simulink model "sampleModel74"  (R2021b)
settings: Solver=VariableStepAuto  StartTime=0.0  StopTime=10.0  RelTol=1e-3
undefined symbols (not defined in the file or in its folder): magnitude, Newton, Raphson
libraries: simulink x10, slpidlib x2
settings Model: Creator=user  LastModifiedBy=user

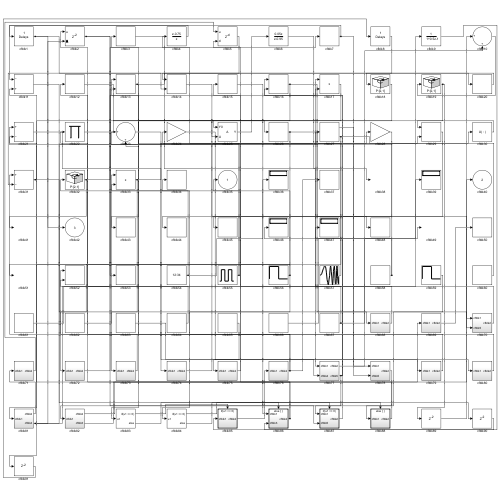
[thumbnail: Simulink's stored preview of the top-level diagram]
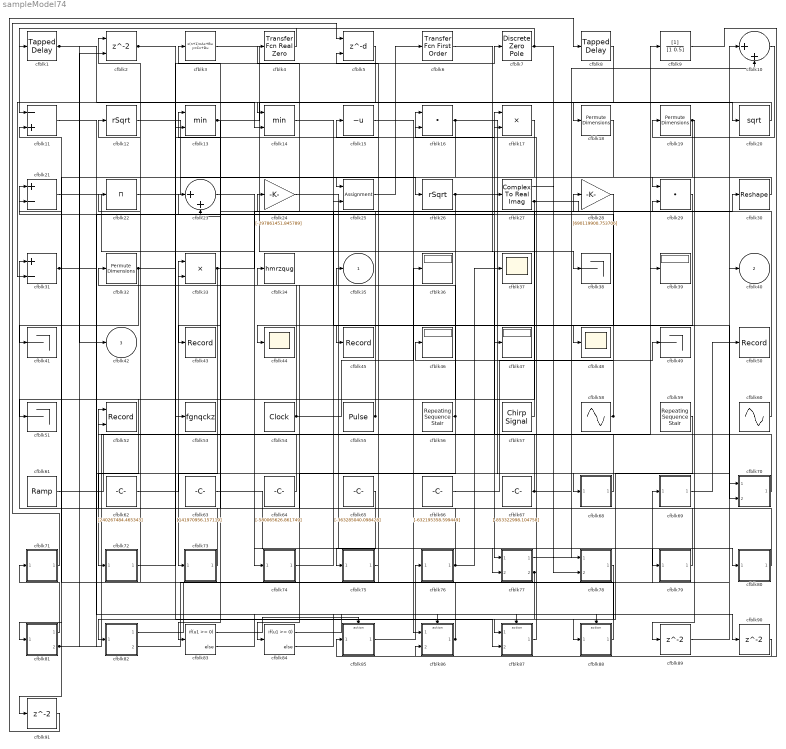
== system sampleModel74 ==
  cfblk1 : simulink/Discrete/Tapped Delay  vinit=0.0  samptime=-1  NumDelays=1  DelayOrder=Oldest  includeCurrent=off
  cfblk10 : Sum  Inputs=|++
  cfblk11 : Sum  Inputs=-+
  cfblk12 : Sqrt  Operator=rSqrt  AlgorithmType=Newton-Raphson  SaturateOnIntegerOverflow=on
  cfblk13 : MinMax  Inputs=2
  cfblk14 : MinMax  Inputs=2
  cfblk15 : UnaryMinus
  cfblk16 : DotProduct  InputSameDT=on  OutDataTypeStr=Inherit: Inherit via internal rule
  cfblk17 : Product
  cfblk18 : PermuteDimensions
  cfblk19 : PermuteDimensions
  cfblk2 : Delay  ShowEnablePort=on  SampleTime=1
      settings: InputPortMap=u0,e6
  cfblk20 : Sqrt  SaturateOnIntegerOverflow=on
  cfblk21 : Sum  Inputs=+-
  cfblk22 : Product  Inputs=*
  cfblk23 : Sum  Inputs=|++
  cfblk24 : Gain  Gain=[-297861451.845789]
  cfblk25 : Assignment  DiagnosticForDimensions=Warning  IndexOptions=Index vector (dialog)  Indices=1  OutputSizes=1
  cfblk26 : Sqrt  Operator=rSqrt  AlgorithmType=Newton-Raphson  SaturateOnIntegerOverflow=on
  cfblk27 : ComplexToRealImag
  cfblk28 : Gain  Gain=[690119900.753706]
  cfblk29 : DotProduct  InputSameDT=on  OutDataTypeStr=Inherit: Inherit via internal rule
  cfblk3 : DiscreteStateSpace
  cfblk30 : Reshape
  cfblk31 : Sum  Inputs=+-
  cfblk32 : PermuteDimensions
  cfblk33 : Product  Inputs=**
  cfblk34 : ToWorkspace  VariableName=hmrzqug  SaveFormat=Timeseries  SampleTime=-1
  cfblk{36,39,46..47} (4 alike) : Display
  cfblk37 : Scope
  cfblk{38,41,49,51} (4 alike) : Terminator
  cfblk4 : simulink/Discrete/Transfer Fcn Real Zero  ZeroZ=0.75  ICPrevInput=0.0  DoSatur=off
      settings: SourceProductBaseCode=SL
  cfblk43 : Record  FileSettingsInternal="{\"entries\":[{\"content\":{\"excelSettings\":{\"content\":{},\"type\":\"Streamout.ExcelSettings\"}},\"type\":\"Streamout.FileSettingStorage\",\"uuid\":\"48ba1b95-7696-4fb7-898a-d0dd139d0650\"}],\"packageUris\":[\"http://schema.mathworks.com/mf0/streamout_blocks/R2020a\"],\"version\":\"1.0\"}"  SignalsInternal="{\"entries\":[{\"content\":{\"signals\":[{\"content\":{\"blockPath\":[\"sampleModel74/cfblk43\"],\"channel\":[],\"dimensions\":[1,1],\"domain\":\"sampleModel74/cfblk43\",\"lineColor\":\"#edb120\",\"plots\":[1],\"port\":1,\"sid\":[\"\"],\"signalID\":2737,\"signalName\":\"cfblk17\"},\"type\":\"RecordBlkView.Signal\",\"uuid\":\"e86d3584-fb59-4afd-a1db-0bd2ffc62248\"}]},\"type\":\"RecordBlkView.InputSignals\",\"uuid\":\"38ef3183-be6e-4a9e-be3e-a4fb90b5b1f9\"}],\"packageUris\":[\"http://schema.mathworks.com/mf0/streamout_blocks/R2020a\"],\"version\":\"1.0\"}"  VisualizationBindings="{\"sparklinesplugin\":{\"info\":[{\"bindingParametersList\":[],\"subplotID\":1}]}}"
  cfblk44 : Scope
  cfblk45 : Record  FileSettingsInternal="{\"entries\":[{\"content\":{\"excelSettings\":{\"content\":{},\"type\":\"Streamout.ExcelSettings\"}},\"type\":\"Streamout.FileSettingStorage\",\"uuid\":\"c0c04c6a-9287-4ca5-a954-90f3d465e295\"}],\"packageUris\":[\"http://schema.mathworks.com/mf0/streamout_blocks/R2020a\"],\"version\":\"1.0\"}"  SignalsInternal="{\"entries\":[{\"content\":{\"signals\":[{\"content\":{\"blockPath\":[\"sampleModel74/cfblk45\"],\"channel\":[],\"dimensions\":[1],\"domain\":\"sampleModel74/cfblk45\",\"lineColor\":\"#7e2f8e\",\"plots\":[1],\"port\":1,\"sid\":[\"\"],\"signalID\":2741,\"signalName\":\"cfblk28\"},\"type\":\"RecordBlkView.Signal\",\"uuid\":\"fff33049-bbd2-4e7c-9b44-5c2925b8b3c0\"}]},\"type\":\"RecordBlkView.InputSignals\",\"uuid\":\"e4e584d3-6e89-4657-a415-00abe31742ed\"}],\"packageUris\":[\"http://schema.mathworks.com/mf0/streamout_blocks/R2020a\"],\"version\":\"1.0\"}"  VisualizationBindings="{\"sparklinesplugin\":{\"info\":[{\"bindingParametersList\":[],\"subplotID\":1}]}}"
  cfblk48 : Scope
  cfblk5 : Delay  DelayLengthSource=Input port  SampleTime=1
      settings: InputPortMap=u0,p1
  cfblk50 : Record  FileSettingsInternal="{\"entries\":[{\"content\":{\"excelSettings\":{\"content\":{},\"type\":\"Streamout.ExcelSettings\"}},\"type\":\"Streamout.FileSettingStorage\",\"uuid\":\"2063bf91-ee10-44c6-85e7-3db64ce144e7\"}],\"packageUris\":[\"http://schema.mathworks.com/mf0/streamout_blocks/R2020a\"],\"version\":\"1.0\"}"  SignalsInternal="{\"entries\":[{\"content\":{\"signals\":[{\"content\":{\"blockPath\":[\"sampleModel74/cfblk50\"],\"channel\":[],\"dimensions\":[1],\"domain\":\"sampleModel74/cfblk50\",\"lineColor\":\"#77ac30\",\"plots\":[1],\"port\":1,\"sid\":[\"\"],\"signalID\":2745,\"signalName\":\"cfblk69\"},\"type\":\"RecordBlkView.Signal\",\"uuid\":\"c73e1d6d-ec7e-4053-a185-d07a06e2b1ae\"}]},\"type\":\"RecordBlkView.InputSignals\",\"uuid\":\"2d8ce3cf-72b1-4d47-bc01-c7806f849a67\"}],\"packageUris\":[\"http://schema.mathworks.com/mf0/streamout_blocks/R2020a\"],\"version\":\"1.0\"}"  VisualizationBindings="{\"sparklinesplugin\":{\"info\":[{\"bindingParametersList\":[],\"subplotID\":1}]}}"
  cfblk52 : Record  FileSettingsInternal="{\"entries\":[{\"content\":{\"excelSettings\":{\"content\":{},\"type\":\"Streamout.ExcelSettings\"}},\"type\":\"Streamout.FileSettingStorage\",\"uuid\":\"a33d63da-2fbc-4813-9a5f-8919b3ff38c5\"}],\"packageUris\":[\"http://schema.mathworks.com/mf0/streamout_blocks/R2020a\"],\"version\":\"1.0\"}"  Layout=[1 1]  SignalsInternal="{\"entries\":[{\"content\":{\"signals\":[{\"content\":{\"blockPath\":[\"sampleModel74/cfblk52\"],\"channel\":[],\"dimensions\":[1],\"domain\":\"sampleModel74/cfblk52\",\"lineColor\":\"#a2142f\",\"plots\":[1],\"port\":1,\"sid\":[\"\"],\"signalID\":2749,\"signalName\":\"cfblk73\"},\"type\":\"RecordBlkView.Signal\",\"uuid\":\"3106f9a6-1d98-4c48-b4a9-0628818cd6a2\"},{\"content\":{\"blockPath\":[\"sampleModel74/cfblk52\"],\"channel\":[],\"dimensions\":[1],\"domain\":\"sampleModel74/cfblk52\",\"lineColor\":\"#139fff\",\"plots\":[1],\"port\":2,\"sid\":[\"\"],\"signalID\":2753,\"signalName\":\"cfblk64\"},\"type\":\"RecordBlkView.Signal\",\"uuid\":\"3007701b-6436-4cea-b82a-5ba8fd36c4e2\"}]},\"type\":\"RecordBlkView.InputSignals\",\"uuid\":\"9f57cf0e-22d1-4040-b944-b37ea4da367a\"}],\"packageUris\":[\"http://schema.mathworks.com/mf0/streamout_blocks/R2020a\"],\"version\":\"1.0\"}"  VisualizationBindings="{\"xyplotplugin\":{\"info\":[{\"series\":[{\"bindingParametersList\":[{\"parameter\":\"X-Axis\",\"signalID\":2749,\"signalName\":\"cfblk73\"},{\"parameter\":\"Y-Axis\",\"signalID\":2753,\"signalName\":\"cfblk64\"}],\"seriesID\":56445}],\"subplotID\":1}]}}"  CompatibilityTag=XY
  cfblk53 : ToWorkspace  VariableName=fgnqckz  SaveFormat=Timeseries  SampleTime=-1
  cfblk54 : DigitalClock
  cfblk55 : DiscretePulseGenerator  PulseType=Time based  Amplitude=[301093662.355844]  Period=[78291214.877593]  PulseWidth=5  PhaseDelay=[1.000000]
  cfblk56 : simulink/Sources/Repeating Sequence Stair  OutValues=[-38877685.461158, -866960158.323522]  tsamp=-1  OutMin=[]  OutMax=[]  OutDataTypeStr=double  OutputDataTypeScalingMode=double  OutDataType=fixdt(0,8)  ConRadixGroup=Best Precision: Vector-wise  OutScaling=2^-12
  cfblk57 : simulink/Sources/Chirp Signal  f1=[-130713625.876900]  T=[92266406.941991]  f2=[714551221.409625]
  cfblk58 : Sin  Amplitude=[-215573379.116947]  Bias=[658746098.891417]  SampleTime=0
  cfblk59 : simulink/Sources/Repeating Sequence Stair  OutValues=[-482847382.722123, -898676029.322696]  tsamp=-1  OutMin=[]  OutMax=[]  OutDataTypeStr=double  OutputDataTypeScalingMode=double  OutDataType=fixdt(0,8)  ConRadixGroup=Best Precision: Vector-wise  OutScaling=2^-12
  cfblk6 : simulink/Discrete/Transfer Fcn First Order  PoleZ=0.95  ICPrevOutput=0.0  DoSatur=off
  cfblk60 : Sin  Amplitude=[827954509.071652]  Bias=[417393928.339158]  SampleTime=0
  cfblk61 : simulink/Sources/Ramp  slope=[3672.630180]  start=[38.252533]  InitialOutput=[-938336.900996]
  cfblk62 : Constant  Value=[240267484.465343]  SampleTime=1
  cfblk63 : Constant  Value=[141970956.157119]  SampleTime=1
  cfblk64 : Constant  Value=[-580065626.861749]  SampleTime=1
  cfblk65 : Constant  Value=[-363285040.098428]  SampleTime=1
  cfblk66 : Constant  Value=[-632195358.599449]  SampleTime=1
  cfblk67 : Constant  Value=[-853322998.104758]  SampleTime=1
  cfblk68 : Subsystem
  cfblk69 : Subsystem
  cfblk7 : DiscreteZeroPole  Poles=[0 0.5]  Gain=1
  cfblk70 : Subsystem
  cfblk71 : Subsystem
  cfblk72 : Subsystem
  cfblk73 : Subsystem
  cfblk74 : Subsystem
  cfblk75 : Subsystem
  cfblk76 : Subsystem
  cfblk77 : Subsystem
  cfblk78 : Subsystem
  cfblk79 : Subsystem
  cfblk8 : simulink/Discrete/Tapped Delay  vinit=0.0  samptime=-1  NumDelays=1  DelayOrder=Oldest  includeCurrent=off
  cfblk80 : Subsystem
  cfblk81 : Subsystem
  cfblk82 : Subsystem
  cfblk83 : If  IfExpression=u1 >= 0  SampleTime=1
  cfblk84 : If  IfExpression=u1 >= 0  SampleTime=1
  cfblk85 : Subsystem  TreatAsAtomicUnit=on
  cfblk86 : Subsystem  TreatAsAtomicUnit=on
  cfblk87 : Subsystem  TreatAsAtomicUnit=on
  cfblk88 : Subsystem  TreatAsAtomicUnit=on
  cfblk89 : Delay  SampleTime=1
  cfblk9 : DiscreteFilter  SampleTime=1
  cfblk90 : Delay  SampleTime=1
  cfblk91 : Delay  SampleTime=1
  cfblk35 : Outport
  cfblk40 : Outport  Port=2
  cfblk42 : Outport  Port=3
  wires:
  cfblk25/1 -> cfblk6/1
  cfblk54/1 -> cfblk32/1, cfblk36/1
  cfblk82/1(cfblk2) -> cfblk69/1(cfblk1)
  cfblk73/1(cfblk2) -> cfblk52/1
  cfblk3/1 -> cfblk77/1(cfblk1)
  cfblk27/1 -> cfblk78/1(cfblk1)
  cfblk1/1 -> cfblk42/1, cfblk14/2
  cfblk33/1 -> cfblk73/1(cfblk1), cfblk29/2
  cfblk57/1 -> cfblk24/1
  cfblk65/1 -> cfblk75/1(cfblk1)
  cfblk85/1(cfblk2) -> cfblk76/1(cfblk1)
  cfblk29/1 -> cfblk44/1
  cfblk16/1 -> cfblk68/1(cfblk1), cfblk83/1
  cfblk74/1(cfblk2) -> cfblk28/1
  cfblk64/1 -> cfblk52/2
  cfblk12/1 -> cfblk25/1
  cfblk76/1(cfblk2) -> cfblk31/1, cfblk34/1, cfblk37/1
  cfblk4/1 -> cfblk11/1
  cfblk23/1 -> cfblk77/2(cfblk4)
  cfblk75/1(cfblk2) -> cfblk15/1
  cfblk21/1 -> cfblk74/1(cfblk1)
  cfblk67/1 -> cfblk49/1, cfblk5/2
  cfblk13/1 -> cfblk20/1, cfblk23/2
  cfblk10/1 -> cfblk19/1
  cfblk8/1 -> cfblk18/1
  cfblk66/1 -> cfblk39/1
  cfblk56/1 -> cfblk33/1, cfblk84/1, cfblk51/1
  cfblk15/1 -> cfblk86/1(cfblk1)
  cfblk24/1 -> cfblk80/1(cfblk1)
  cfblk58/1 -> cfblk46/1, cfblk23/1
  cfblk55/1 -> cfblk4/1, cfblk21/2
  cfblk28/1 -> cfblk45/1
  cfblk68/1(cfblk2) -> cfblk17/1
  cfblk27/2 -> cfblk30/1, cfblk72/1(cfblk1)
  cfblk60/1 -> cfblk3/1
  cfblk87/1(cfblk2) -> cfblk47/1
  cfblk81/1(cfblk2) -> cfblk71/1(cfblk1)
  cfblk62/1 -> cfblk33/2
  cfblk17/1 -> cfblk43/1
  cfblk19/1 -> cfblk25/2, cfblk89/1
  cfblk20/1 -> cfblk14/1
  cfblk79/1(cfblk2) -> cfblk13/1
  cfblk5/1 -> cfblk31/2
  cfblk71/1(cfblk2) -> cfblk5/1
  cfblk61/1 -> cfblk9/1
  cfblk14/1 -> cfblk48/1
  cfblk78/1(cfblk2) -> cfblk87/1(cfblk1)
  cfblk22/1 -> cfblk26/1
  cfblk31/1 -> cfblk11/2, cfblk90/1
  cfblk7/1 -> cfblk1/1, cfblk78/2(cfblk5)
  cfblk69/1(cfblk2) -> cfblk50/1
  cfblk32/1 -> cfblk17/2, cfblk41/1
  cfblk81/2(cfblk4) -> cfblk13/2, cfblk27/1, cfblk2/2
  cfblk63/1 -> cfblk79/1(cfblk1)
  cfblk72/1(cfblk2) -> cfblk7/1
  cfblk59/1 -> cfblk88/1(cfblk1)
  cfblk88/1(cfblk2) -> cfblk35/1
  cfblk26/1 -> cfblk70/1(cfblk1), cfblk81/1(cfblk1)
  cfblk70/1(cfblk2) -> cfblk2/1
  cfblk2/1 -> cfblk53/1, cfblk87/2(cfblk5)
  cfblk77/1(cfblk2) -> cfblk10/2
  cfblk30/1 -> cfblk29/1
  cfblk6/1 -> cfblk38/1
  cfblk82/2(cfblk3) -> cfblk40/1
  cfblk80/1(cfblk2) -> cfblk22/1
  cfblk86/1(cfblk2) -> cfblk12/1, cfblk21/1
  cfblk77/2(cfblk5) -> cfblk82/1(cfblk1), cfblk16/1, cfblk16/2
  cfblk9/1 -> cfblk86/2(cfblk3)
  cfblk11/1 -> cfblk70/2(cfblk5)
  cfblk83/1 -> cfblk85/Action
  cfblk83/2 -> cfblk86/Action
  cfblk84/1 -> cfblk87/Action
  cfblk84/2 -> cfblk88/Action
  cfblk89/1 -> cfblk10/1
  cfblk90/1 -> cfblk85/1(cfblk1)
  cfblk18/1 -> cfblk91/1
  cfblk91/1 -> cfblk8/1

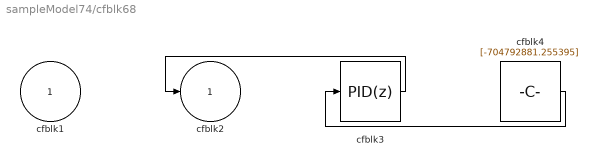
== system sampleModel74/cfblk68 ==
  cfblk1 : Inport
  cfblk3 : slpidlib/PID Controller  Controller=PID  Form=Parallel  TimeDomain=Discrete-time  UseExternalTs=off  SampleTime=1  IntegratorMethod=Forward Euler  FilterMethod=Forward Euler  ControllerParametersSource=internal  P=1  I=1  D=0  UseFilter=on  N=100  TunerSelectOption=Transfer Function Based (PID Tuner App)  InitialConditionSource=internal  InitialConditionForIntegrator=0  InitialConditionForFilter=0  DifferentiatorICPrevScaledInput=0  ExternalReset=none  TrackingMode=off  Kt=1  LimitOutput=off  SatLimitsSource=internal  UpperSaturationLimit=inf  LowerSaturationLimit=-inf  LinearizeAsGain=off  AntiWindupMode=none  Kb=1  POutMin=[]  POutMax=[]  IOutMin=[]  IOutMax=[]  DOutMin=[]  DOutMax=[]  NOutMin=[]  NOutMax=[]  SumOutMin=[]  SumOutMax=[]  SaturationOutMin=[]  SaturationOutMax=[]  PParamMin=[]  PParamMax=[]  IParamMin=[]  IParamMax=[]  DParamMin=[]  DParamMax=[]  NParamMin=[]  NParamMax=[]  KbParamMin=[]  KbParamMax=[]  KtParamMin=[]  KtParamMax=[]  KbOutMin=[]  KbOutMax=[]  KtOutMin=[]  KtOutMax=[]  IntegratorOutMin=[]  IntegratorOutMax=[]  FilterOutMin=[]  FilterOutMax=[]  SumI1OutMin=[]  SumI1OutMax=[]  SumI2OutMin=[]  SumI2OutMax=[]  SumI3OutMin=[]  SumI3OutMax=[]  SumI4OutMin=[]  SumI4OutMax=[]  SumDOutMin=[]  SumDOutMax=[]  DifferentiatorOutMin=[]  DifferentiatorOutMax=[]  FilterDiffOutCoefMin=[]  FilterDiffOutCoefMax=[]  ReciprocalOutMin=[]  ReciprocalOutMax=[]  SumDenOutMin=[]  SumDenOutMax=[]  SumNumOutMin=[]  SumNumOutMax=[]  DivideOutMin=[]  DivideOutMax=[]  UdiffTsProdOutMin=[]  UdiffTsProdOutMax=[]  NTsProdOutMin=[]  NTsProdOutMax=[]  UintegralTsProdOutMin=[]  UintegralTsProdOutMax=[]  UngainTsProdOutMin=[]  UngainTsProdOutMax=[]  IntegratorContinuousStateAttributes=''  IntegratorStateMustResolveToSignalObject=off  IntegratorRTWStateStorageClass=Auto  FilterContinuousStateAttributes=''  FilterStateMustResolveToSignalObject=off  FilterRTWStateStorageClass=Auto  ParallelPVariant=InternalParameters  IdealPVariant=Disabled  IVariant=InternalParameters  DVariant=InternalParameters  IntegratorVariant=Discrete  SatVariant=Disabled  AWVariant=Passthrough  PCopyVariant=Disabled  TRVariant=Disabled  FdbkBlocksVariant=Forward  IdealPFdbkVariant=Disabled  SatFdbkVariant=Disabled  DerivativeFilterVariant=ForwardEulerFilter  NVariant=InternalParameters  NCopyVariant=Disabled  FilterICVariant=InternalICsFilter  IntegratorICVariant=InternalICs  ExternalResetVariant=Disabled  TRSumVariant=Passthrough  SumFdbkVariant=Disabled  SumVariant=Sum_PID  TsampFilterVariant=InternalTs  TsampNgainVariant=Passthrough  TsampIntegralVariant=Passthrough  ExternalSaturationOutDataTypeStr=Inherit: Same as second input
  cfblk4 : Constant  Value=[-704792881.255395]  SampleTime=1
  cfblk2 : Outport
  wires:
  cfblk3/1 -> cfblk2/1
  cfblk4/1 -> cfblk3/1

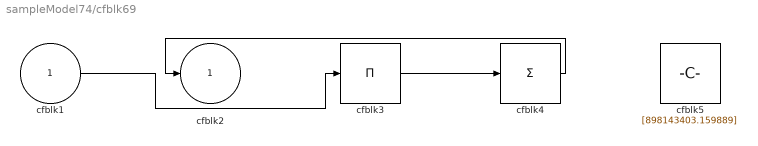
== system sampleModel74/cfblk69 ==
  cfblk1 : Inport
  cfblk3 : Product  Inputs=*
  cfblk4 : Sum  Inputs=+
  cfblk5 : Constant  Value=[898143403.159889]  SampleTime=1
  cfblk2 : Outport
  wires:
  cfblk3/1 -> cfblk4/1
  cfblk4/1 -> cfblk2/1
  cfblk1/1 -> cfblk3/1

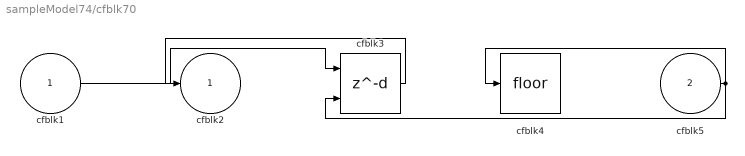
== system sampleModel74/cfblk70 ==
  cfblk1 : Inport
  cfblk5 : Inport  Port=2
  cfblk3 : Delay  DelayLengthSource=Input port  SampleTime=1
      settings: InputPortMap=u0,p1
  cfblk4 : Rounding
  cfblk2 : Outport
  wires:
  cfblk1/1 -> cfblk3/1
  cfblk5/1 -> cfblk3/2, cfblk4/1
  cfblk3/1 -> cfblk2/1

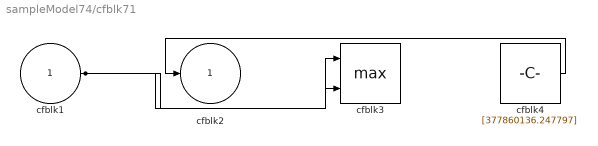
== system sampleModel74/cfblk71 ==
  cfblk1 : Inport
  cfblk3 : MinMax  Function=max  Inputs=2
  cfblk4 : Constant  Value=[377860136.247797]  SampleTime=1
  cfblk2 : Outport
  wires:
  cfblk4/1 -> cfblk2/1
  cfblk1/1 -> cfblk3/1, cfblk3/2

== system sampleModel74/cfblk72 ==
  cfblk1 : Inport
  cfblk3 : Constant  Value=[711047565.909843]  SampleTime=1
  cfblk2 : Outport
  wires:
  cfblk1/1 -> cfblk2/1

== system sampleModel74/cfblk73 ==
  cfblk1 : Inport
  cfblk3 : Constant  Value=[885206688.060875]  SampleTime=1
  cfblk2 : Outport
  wires:
  cfblk1/1 -> cfblk2/1

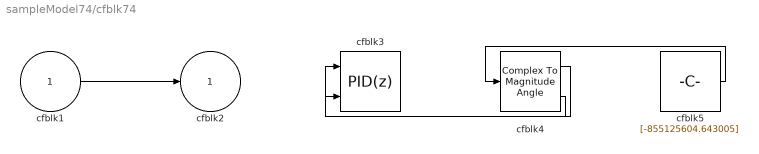
== system sampleModel74/cfblk74 ==
  cfblk1 : Inport
  cfblk3 : slpidlib/PID Controller (2DOF)  Controller=PID  Form=Parallel  TimeDomain=Discrete-time  UseExternalTs=off  SampleTime=1  IntegratorMethod=Forward Euler  FilterMethod=Forward Euler  ControllerParametersSource=internal  P=1  I=1  D=0  UseFilter=on  N=100  b=1  c=1  TunerSelectOption=Transfer Function Based (PID Tuner App)  InitialConditionSource=internal  InitialConditionForIntegrator=0  InitialConditionForFilter=0  DifferentiatorICPrevScaledInput=0  ExternalReset=none  TrackingMode=off  Kt=1  LimitOutput=off  SatLimitsSource=internal  UpperSaturationLimit=inf  LowerSaturationLimit=-inf  LinearizeAsGain=off  AntiWindupMode=none  Kb=1  POutMin=[]  POutMax=[]  IOutMin=[]  IOutMax=[]  DOutMin=[]  DOutMax=[]  NOutMin=[]  NOutMax=[]  bOutMin=[]  bOutMax=[]  cOutMin=[]  cOutMax=[]  SumOutMin=[]  SumOutMax=[]  SaturationOutMin=[]  SaturationOutMax=[]  PParamMin=[]  PParamMax=[]  IParamMin=[]  IParamMax=[]  DParamMin=[]  DParamMax=[]  NParamMin=[]  NParamMax=[]  bParamMin=[]  bParamMax=[]  cParamMin=[]  cParamMax=[]  KbParamMin=[]  KbParamMax=[]  KtParamMin=[]  KtParamMax=[]  KbOutMin=[]  KbOutMax=[]  KtOutMin=[]  KtOutMax=[]  IntegratorOutMin=[]  IntegratorOutMax=[]  FilterOutMin=[]  FilterOutMax=[]  SumI1OutMin=[]  SumI1OutMax=[]  SumI2OutMin=[]  SumI2OutMax=[]  SumI3OutMin=[]  SumI3OutMax=[]  SumI4OutMin=[]  SumI4OutMax=[]  SumDOutMin=[]  SumDOutMax=[]  Sum1OutMin=[]  Sum1OutMax=[]  Sum2OutMin=[]  Sum2OutMax=[]  Sum3OutMin=[]  Sum3OutMax=[]  DifferentiatorOutMin=[]  DifferentiatorOutMax=[]  FilterDiffOutCoefMin=[]  FilterDiffOutCoefMax=[]  ReciprocalOutMin=[]  ReciprocalOutMax=[]  SumDenOutMin=[]  SumDenOutMax=[]  SumNumOutMin=[]  SumNumOutMax=[]  DivideOutMin=[]  DivideOutMax=[]  UdiffTsProdOutMin=[]  UdiffTsProdOutMax=[]  NTsProdOutMin=[]  NTsProdOutMax=[]  UintegralTsProdOutMin=[]  UintegralTsProdOutMax=[]  UngainTsProdOutMin=[]  UngainTsProdOutMax=[]  IntegratorContinuousStateAttributes=''  IntegratorStateMustResolveToSignalObject=off  IntegratorRTWStateStorageClass=Auto  FilterContinuousStateAttributes=''  FilterStateMustResolveToSignalObject=off  FilterRTWStateStorageClass=Auto  ParallelPVariant=InternalParameters  IdealPVariant=Disabled  IVariant=InternalParameters  DVariant=InternalParameters  bVariant=InternalParameters  cVariant=InternalParameters  IntegratorVariant=Discrete  SatVariant=Disabled  AWVariant=Passthrough  PCopyVariant=Disabled  TRVariant=Disabled  FdbkBlocksVariant=Forward  IdealPFdbkVariant=Disabled  SatFdbkVariant=Disabled  DerivativeFilterVariant=ForwardEulerFilter  NVariant=InternalParameters  NCopyVariant=Disabled  FilterICVariant=InternalICsFilter  IntegratorICVariant=InternalICs  ExternalResetVariant=Disabled  TRSumVariant=Passthrough  SumFdbkVariant=Disabled  SumVariant=Sum_PID  TsampFilterVariant=InternalTs  TsampNgainVariant=Passthrough  TsampIntegralVariant=Passthrough  ExternalSaturationOutDataTypeStr=Inherit: Same as second input
      settings: SourceProductBaseCode=SL
  cfblk4 : ComplexToMagnitudeAngle
  cfblk5 : Constant  Value=[-855125604.643005]  SampleTime=1
  cfblk2 : Outport
  wires:
  cfblk1/1 -> cfblk2/1
  cfblk5/1 -> cfblk4/1
  cfblk4/1 -> cfblk3/1
  cfblk4/2 -> cfblk3/2

== system sampleModel74/cfblk75 ==
  cfblk1 : Inport
  cfblk3 : DiscreteStateSpace
  cfblk4 : Math  Operator=magnitude^2  SaturateOnIntegerOverflow=on
  cfblk2 : Outport
  wires:
  cfblk1/1 -> cfblk3/1
  cfblk3/1 -> cfblk4/1
  cfblk4/1 -> cfblk2/1

== system sampleModel74/cfblk76 ==
  cfblk1 : Inport
  cfblk3 : Rounding
  cfblk2 : Outport
  wires:
  cfblk3/1 -> cfblk2/1
  cfblk1/1 -> cfblk3/1

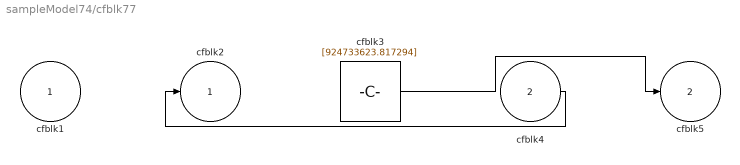
== system sampleModel74/cfblk77 ==
  cfblk1 : Inport
  cfblk4 : Inport  Port=2
  cfblk3 : Constant  Value=[924733623.817294]  SampleTime=1
  cfblk2 : Outport
  cfblk5 : Outport  Port=2
  wires:
  cfblk3/1 -> cfblk5/1
  cfblk4/1 -> cfblk2/1

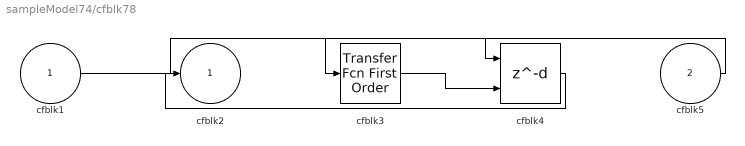
== system sampleModel74/cfblk78 ==
  cfblk1 : Inport
  cfblk5 : Inport  Port=2
  cfblk3 : simulink/Discrete/Transfer Fcn First Order  PoleZ=0.95  ICPrevOutput=0.0  DoSatur=off
  cfblk4 : Delay  DelayLengthSource=Input port  SampleTime=1
      settings: InputPortMap=u0,p1
  cfblk2 : Outport
  wires:
  cfblk1/1 -> cfblk4/1
  cfblk4/1 -> cfblk2/1
  cfblk3/1 -> cfblk4/2
  cfblk5/1 -> cfblk3/1

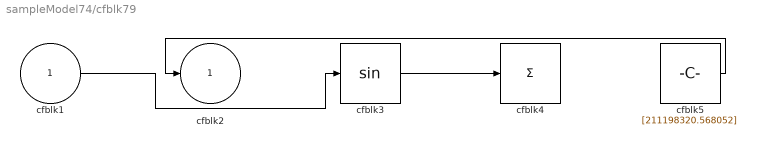
== system sampleModel74/cfblk79 ==
  cfblk1 : Inport
  cfblk3 : Trigonometry
  cfblk4 : Sum  Inputs=+
  cfblk5 : Constant  Value=[211198320.568052]  SampleTime=1
  cfblk2 : Outport
  wires:
  cfblk5/1 -> cfblk2/1
  cfblk1/1 -> cfblk3/1
  cfblk3/1 -> cfblk4/1

== system sampleModel74/cfblk80 ==
  cfblk1 : Inport
  cfblk3 : simulink/Discrete/Tapped Delay  vinit=0.0  samptime=-1  NumDelays=1  DelayOrder=Oldest  includeCurrent=off
  cfblk4 : Constant  Value=[-523758652.321392]  SampleTime=1
  cfblk2 : Outport
  wires:
  cfblk1/1 -> cfblk3/1
  cfblk3/1 -> cfblk2/1

== system sampleModel74/cfblk81 ==
  cfblk1 : Inport
  cfblk3 : PermuteDimensions
  cfblk2 : Outport
  cfblk4 : Outport  Port=2
  wires:
  cfblk1/1 -> cfblk3/1
  cfblk3/1 -> cfblk4/1, cfblk2/1

== system sampleModel74/cfblk82 ==
  cfblk1 : Inport
  cfblk2 : Outport
  cfblk3 : Outport  Port=2
  wires:
  cfblk1/1 -> cfblk3/1, cfblk2/1

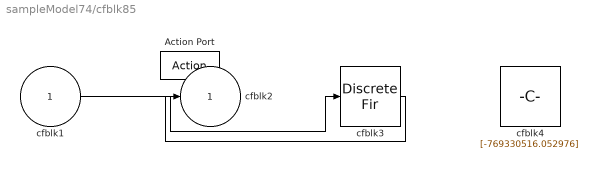
== system sampleModel74/cfblk85 ==
  cfblk1 : Inport
  Action Port : ActionPort  ActionPortLabel=if(u1 >= 0)
  cfblk3 : DiscreteFir
  cfblk4 : Constant  Value=[-769330516.052976]  SampleTime=1
  cfblk2 : Outport
  wires:
  cfblk1/1 -> cfblk3/1
  cfblk3/1 -> cfblk2/1

== system sampleModel74/cfblk86 ==
  cfblk1 : Inport
  cfblk3 : Inport  Port=2
  Action Port : ActionPort  ActionPortLabel=else
  cfblk2 : Outport
  wires:
  cfblk1/1 -> cfblk2/1

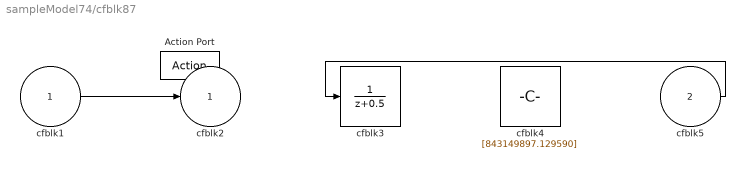
== system sampleModel74/cfblk87 ==
  cfblk1 : Inport
  cfblk5 : Inport  Port=2
  Action Port : ActionPort  ActionPortLabel=if(u1 >= 0)
  cfblk3 : DiscreteTransferFcn
  cfblk4 : Constant  Value=[843149897.129590]  SampleTime=1
  cfblk2 : Outport
  wires:
  cfblk1/1 -> cfblk2/1
  cfblk5/1 -> cfblk3/1

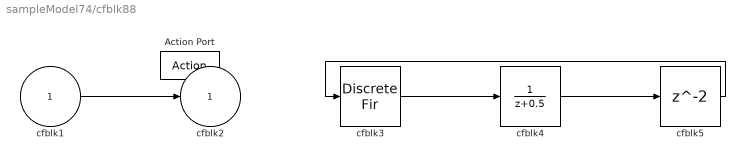
== system sampleModel74/cfblk88 ==
  cfblk1 : Inport
  Action Port : ActionPort  ActionPortLabel=else
  cfblk3 : DiscreteFir
  cfblk4 : DiscreteTransferFcn
  cfblk5 : Delay
  cfblk2 : Outport
  wires:
  cfblk3/1 -> cfblk4/1
  cfblk1/1 -> cfblk2/1
  cfblk4/1 -> cfblk5/1
  cfblk5/1 -> cfblk3/1
